simulink model "model"  (R2014a)
(part 5 of 5)

  powergui : powerlib/powergui  Priority=1  SimulationMode=Continuous  SolverType=Tustin  SampleTime=50e-6  frequency=60  SPID=off  DisableSnubberDevices=off  DisableRonSwitches=off  DisableVfSwitches=off  SwTol=0  Interpol=off  DisplayEquations=off  Ts=0  methode=off  frequencyindice=60  Pbase=100e6  ErrMax=1e-4  Iterations=50  UnitsV=kV  UnitsW=MW  FunctionMessages=off  echomessages=off  HookPort=off  EnableUseOfTLC=off  x0status=blocks  RestoreLinks=warning  ResistiveCurrentMeasurement=off  Frange=[0:2:500]  Ylog=off  Xlog=on  ShowGrid=off  save=off  variable=ZData  structure=0  ZoomFFT=off  StartTime=0.0  cycles=1  DisplayStyle=1  fundamental=60  FreqAxis=off  MaxFrequency=1000  frequencyindicesteady=1  RmsSteady=1  display=off
  Ötztal___Zirl_CN_147563007_110000_CN_100404264_110000 : powerlib/Elements/Distributed Parameters Line  Phases=3  Frequency=60  Resistance=[0.01273 0.3864]  Inductance="[0.9337e-3  4.1264e-3]"  Capacitance=[12.74e-9 7.751e-9]  Length=100  x1=[0 0 0 0; 0.0001244 0 0 0; 0.0002488 0 0 0; 0.0003733 0 0 0; 0.0004977 0 0 0; 0.0006221 0 0 0]  x2=[0 0 0 0; 0.0001244 0 0 0; 0.0002488 0 0 0; 0.0003733 0 0 0; 0.0004977 0 0 0; 0.0006221 0 0 0]  x3=[0 0 0 0; 0.0001244 0 0 0; 0.0002488 0 0 0; 0.0003733 0 0 0; 0.0004977 0 0 0; 0.0006221 0 0 0]  x4=[0 0 0 0; 0.0001244 0 0 0; 0.0002488 0 0 0; 0.0003733 0 0 0; 0.0004977 0 0 0; 0.0006221 0 0 0]  x5=0  V1=ones(3,3)  V2=ones(3,3)  I1=ones(3,3)  I2=ones(3,3)  nHarmo=1  Measurements=None
  connections:
  _CN_403466241_230000_CN_403481611_230000/LConn1 -- T_403466241__/LConn1 -- _CN_403466241_230000_CN_401936547_230000/LConn1
  _CN_403466241_230000_CN_403481611_230000/LConn2 -- T_403466241__/LConn2 -- _CN_403466241_230000_CN_401936547_230000/LConn2
  _CN_403466241_230000_CN_403481611_230000/LConn3 -- T_403466241__/LConn3 -- _CN_403466241_230000_CN_401936547_230000/LConn3 -- bus1/LConn1
  _CN_403466241_230000_CN_403481611_230000/RConn1 -- T_403481611__/LConn1 -- _CN_403481611_230000_CN_252757805_230000/LConn1 -- _CN_403481611_230000_CN_381823435_230000/LConn1
  _CN_403466241_230000_CN_403481611_230000/RConn2 -- T_403481611__/LConn2 -- _CN_403481611_230000_CN_252757805_230000/LConn2 -- _CN_403481611_230000_CN_381823435_230000/LConn2
  _CN_403466241_230000_CN_403481611_230000/RConn3 -- T_403481611__/LConn3 -- _CN_403481611_230000_CN_252757805_230000/LConn3 -- bus2/LConn1 -- _CN_403481611_230000_CN_381823435_230000/LConn3
  _CN_403466241_230000_CN_401936547_230000/RConn1 -- T_401936547__/RConn1 -- _CN_401936547_230000_CN_254460966_230000/LConn1 -- _CN_401936547_230000_CN_403504849_230000/LConn1 -- L_401936547/LConn1
  _CN_403466241_230000_CN_401936547_230000/RConn2 -- T_401936547__/RConn2 -- _CN_401936547_230000_CN_254460966_230000/LConn2 -- _CN_401936547_230000_CN_403504849_230000/LConn2 -- L_401936547/LConn2
  _CN_403466241_230000_CN_401936547_230000/RConn3 -- T_401936547__/RConn3 -- _CN_401936547_230000_CN_254460966_230000/LConn3 -- _CN_401936547_230000_CN_403504849_230000/LConn3 -- L_401936547/LConn3 -- bus3/LConn1
  _CN_404544820_230000_CN_404544831_230000/LConn1 -- T_404544820__/LConn1 -- _CN_404544820_230000_CN_107789748_230000/LConn1
  _CN_404544820_230000_CN_404544831_230000/LConn2 -- T_404544820__/LConn2 -- _CN_404544820_230000_CN_107789748_230000/LConn2
  _CN_404544820_230000_CN_404544831_230000/LConn3 -- T_404544820__/LConn3 -- _CN_404544820_230000_CN_107789748_230000/LConn3 -- bus4/LConn1
  T_404544831__/LConn1 -- _CN_404544820_230000_CN_404544831_230000/RConn1
  T_404544831__/LConn2 -- _CN_404544820_230000_CN_404544831_230000/RConn2
  _CN_404544820_230000_CN_404544831_230000/RConn3 -- T_404544831__/LConn3 -- bus5/LConn1
  _CN_404544820_230000_CN_107789748_230000/RConn1 -- G_107789748_/RConn1 -- _CN_403525677_230000_CN_107789748_230000/LConn1 -- _CN_296560688_230000_CN_107789748_230000/LConn1
  _CN_404544820_230000_CN_107789748_230000/RConn2 -- G_107789748_/RConn2 -- _CN_403525677_230000_CN_107789748_230000/LConn2 -- _CN_296560688_230000_CN_107789748_230000/LConn2
  _CN_404544820_230000_CN_107789748_230000/RConn3 -- G_107789748_/RConn3 -- _CN_403525677_230000_CN_107789748_230000/LConn3 -- _CN_296560688_230000_CN_107789748_230000/LConn3 -- bus6/LConn1
  _CN_407739530_230000_CN_195977249_230000/LConn1 -- T_407739530__/LConn1 -- _CN_407739530_230000_CN_199773788_230000/LConn1
  _CN_407739530_230000_CN_195977249_230000/LConn2 -- T_407739530__/LConn2 -- _CN_407739530_230000_CN_199773788_230000/LConn2
  _CN_407739530_230000_CN_195977249_230000/LConn3 -- T_407739530__/LConn3 -- _CN_407739530_230000_CN_199773788_230000/LConn3 -- bus7/LConn1
  _CN_407739530_230000_CN_195977249_230000/RConn1 -- T_195977249__สถานีไฟฟ้าแรงสูง_นครชัยศรี/LConn1 -- _CN_195977249_230000_CN_133318523_230000/LConn1
  _CN_407739530_230000_CN_195977249_230000/RConn2 -- T_195977249__สถานีไฟฟ้าแรงสูง_นครชัยศรี/LConn2 -- _CN_195977249_230000_CN_133318523_230000/LConn2
  _CN_407739530_230000_CN_195977249_230000/RConn3 -- T_195977249__สถานีไฟฟ้าแรงสูง_นครชัยศรี/LConn3 -- _CN_195977249_230000_CN_133318523_230000/LConn3 -- bus8/LConn1
  _CN_407739530_230000_CN_199773788_230000/RConn1 -- T_199773788__/LConn1 -- _CN_199773777_230000_CN_199773788_230000/LConn1 -- _CN_199773788_230000_CN_387737843_230000/LConn1 -- _CN_199773788_230000_CN_232344443_230000/LConn1 -- _CN_334185872_230000_CN_199773788_230000/LConn1
  _CN_407739530_230000_CN_199773788_230000/RConn2 -- T_199773788__/LConn2 -- _CN_199773777_230000_CN_199773788_230000/LConn2 -- _CN_199773788_230000_CN_387737843_230000/LConn2 -- _CN_199773788_230000_CN_232344443_230000/LConn2 -- _CN_334185872_230000_CN_199773788_230000/LConn2
  _CN_407739530_230000_CN_199773788_230000/RConn3 -- T_199773788__/LConn3 -- _CN_199773777_230000_CN_199773788_230000/LConn3 -- _CN_199773788_230000_CN_387737843_230000/LConn3 -- _CN_199773788_230000_CN_232344443_230000/LConn3 -- bus9/LConn1 -- _CN_334185872_230000_CN_199773788_230000/LConn3
  _CN_403481611_230000_CN_381823435_230000/RConn1 -- T_381823435__/LConn1 -- _CN_404563246_230000_CN_381823435_230000/LConn1
  _CN_403481611_230000_CN_381823435_230000/RConn2 -- T_381823435__/LConn2 -- _CN_404563246_230000_CN_381823435_230000/LConn2
  _CN_403481611_230000_CN_381823435_230000/RConn3 -- T_381823435__/LConn3 -- _CN_404563246_230000_CN_381823435_230000/LConn3 -- bus10/LConn1
  _CN_403481611_230000_CN_252757805_230000/RConn1 -- T_252757805__/LConn1 -- _CN_254460966_230000_CN_252757805_230000/LConn1
  _CN_403481611_230000_CN_252757805_230000/RConn2 -- T_252757805__/LConn2 -- _CN_254460966_230000_CN_252757805_230000/LConn2
  _CN_403481611_230000_CN_252757805_230000/RConn3 -- T_252757805__/LConn3 -- _CN_254460966_230000_CN_252757805_230000/LConn3 -- bus11/LConn1
  T_403525677__/LConn1 -- _CN_403525677_230000_CN_107789748_230000/RConn1
  T_403525677__/LConn2 -- _CN_403525677_230000_CN_107789748_230000/RConn2
  _CN_403525677_230000_CN_107789748_230000/RConn3 -- T_403525677__/LConn3 -- bus12/LConn1
  _CN_334185872_230000_CN_262815047_230000/LConn1 -- T_334185872__/LConn1 -- _CN_334185872_230000_CN_199773788_230000/RConn1
  _CN_334185872_230000_CN_262815047_230000/LConn2 -- T_334185872__/LConn2 -- _CN_334185872_230000_CN_199773788_230000/RConn2
  _CN_334185872_230000_CN_262815047_230000/LConn3 -- T_334185872__/LConn3 -- _CN_334185872_230000_CN_199773788_230000/RConn3 -- bus13/LConn1
  T_262815047__/LConn1 -- _CN_334185872_230000_CN_262815047_230000/RConn1
  T_262815047__/LConn2 -- _CN_334185872_230000_CN_262815047_230000/RConn2
  _CN_334185872_230000_CN_262815047_230000/RConn3 -- T_262815047__/LConn3 -- bus14/LConn1
  T_404006545__/LConn1 -- _CN_404006545_230000_CN_403692059_230000/LConn1
  T_404006545__/LConn2 -- _CN_404006545_230000_CN_403692059_230000/LConn2
  _CN_404006545_230000_CN_403692059_230000/LConn3 -- T_404006545__/LConn3 -- bus15/LConn1
  _CN_404006545_230000_CN_403692059_230000/RConn1 -- T_403692059__/LConn1 -- _CN_223601302_230000_CN_403692059_230000/LConn1 -- _CN_403692059_230000_CN_155851424_230000/LConn1
  _CN_404006545_230000_CN_403692059_230000/RConn2 -- T_403692059__/LConn2 -- _CN_223601302_230000_CN_403692059_230000/LConn2 -- _CN_403692059_230000_CN_155851424_230000/LConn2
  _CN_404006545_230000_CN_403692059_230000/RConn3 -- T_403692059__/LConn3 -- _CN_223601302_230000_CN_403692059_230000/LConn3 -- _CN_403692059_230000_CN_155851424_230000/LConn3 -- bus16/LConn1
  _CN_250742034_230000_CN_388836605_230000/LConn1 -- T_250742034__/RConn1 -- L_250742034/LConn1
  _CN_250742034_230000_CN_388836605_230000/LConn2 -- T_250742034__/RConn2 -- L_250742034/LConn2
  _CN_250742034_230000_CN_388836605_230000/LConn3 -- T_250742034__/RConn3 -- L_250742034/LConn3 -- bus17/LConn1
  _CN_250742034_230000_CN_388836605_230000/RConn1 -- T_388836605_230000_/LConn1 -- _CN_234182441_230000_CN_388836605_230000/LConn1
  _CN_250742034_230000_CN_388836605_230000/RConn2 -- T_388836605_230000_/LConn2 -- _CN_234182441_230000_CN_388836605_230000/LConn2
  _CN_250742034_230000_CN_388836605_230000/RConn3 -- T_388836605_230000_/LConn3 -- _CN_234182441_230000_CN_388836605_230000/LConn3 -- bus18/LConn1
  T_404291501__/LConn1 -- _CN_404291501_230000_CN_155851424_230000/LConn1
  T_404291501__/LConn2 -- _CN_404291501_230000_CN_155851424_230000/LConn2
  _CN_404291501_230000_CN_155851424_230000/LConn3 -- T_404291501__/LConn3 -- bus19/LConn1
  _CN_404291501_230000_CN_155851424_230000/RConn1 -- G_155851424_Bang_Pakong_Power_Plant/RConn1 -- _CN_345996520_230000_CN_155851424_230000/LConn1 -- _CN_404291513_230000_CN_155851424_230000/LConn1 -- _CN_223601302_230000_CN_155851424_230000/LConn1 -- _CN_403692059_230000_CN_155851424_230000/RConn1
  _CN_404291501_230000_CN_155851424_230000/RConn2 -- G_155851424_Bang_Pakong_Power_Plant/RConn2 -- _CN_345996520_230000_CN_155851424_230000/LConn2 -- _CN_404291513_230000_CN_155851424_230000/LConn2 -- _CN_223601302_230000_CN_155851424_230000/LConn2 -- _CN_403692059_230000_CN_155851424_230000/RConn2
  _CN_404291501_230000_CN_155851424_230000/RConn3 -- G_155851424_Bang_Pakong_Power_Plant/RConn3 -- _CN_345996520_230000_CN_155851424_230000/LConn3 -- bus20/LConn1 -- _CN_404291513_230000_CN_155851424_230000/LConn3 -- _CN_223601302_230000_CN_155851424_230000/LConn3 -- _CN_403692059_230000_CN_155851424_230000/RConn3
  _CN_404563246_230000_CN_176322698_230000/LConn1 -- T_404563246__/LConn1 -- _CN_404563246_230000_CN_404572911_230000/LConn1 -- _CN_404563246_230000_CN_381823435_230000/RConn1
  _CN_404563246_230000_CN_176322698_230000/LConn2 -- T_404563246__/LConn2 -- _CN_404563246_230000_CN_404572911_230000/LConn2 -- _CN_404563246_230000_CN_381823435_230000/RConn2
  _CN_404563246_230000_CN_176322698_230000/LConn3 -- T_404563246__/LConn3 -- _CN_404563246_230000_CN_404572911_230000/LConn3 -- bus21/LConn1 -- _CN_404563246_230000_CN_381823435_230000/RConn3
  _CN_404563246_230000_CN_176322698_230000/RConn1 -- G_176322698_Wang_Noi_Power_Station/RConn1 -- _CN_381823390_230000_CN_176322698_230000/LConn1 -- _CN_401936547_500000_CN_176322698_230000/LConn1 -- _CN_261489769_500000_CN_176322698_230000/LConn1 -- _CN_155847885_500000_CN_176322698_230000/LConn1 -- _CN_199773777_500000_CN_176322698_230000/LConn1 -- _CN_223601302_500000_CN_176322698_230000/LConn1 -- _CN_381823390_500000_CN_176322698_230000/LConn1
  _CN_404563246_230000_CN_176322698_230000/RConn2 -- G_176322698_Wang_Noi_Power_Station/RConn2 -- _CN_381823390_230000_CN_176322698_230000/LConn2 -- _CN_401936547_500000_CN_176322698_230000/LConn2 -- _CN_261489769_500000_CN_176322698_230000/LConn2 -- _CN_155847885_500000_CN_176322698_230000/LConn2 -- _CN_199773777_500000_CN_176322698_230000/LConn2 -- _CN_223601302_500000_CN_176322698_230000/LConn2 -- _CN_381823390_500000_CN_176322698_230000/LConn2
  _CN_404563246_230000_CN_176322698_230000/RConn3 -- G_176322698_Wang_Noi_Power_Station/RConn3 -- _CN_381823390_230000_CN_176322698_230000/LConn3 -- _CN_401936547_500000_CN_176322698_230000/LConn3 -- _CN_261489769_500000_CN_176322698_230000/LConn3 -- _CN_155847885_500000_CN_176322698_230000/LConn3 -- _CN_199773777_500000_CN_176322698_230000/LConn3 -- _CN_223601302_500000_CN_176322698_230000/LConn3 -- _CN_381823390_500000_CN_176322698_230000/LConn3 -- bus22/LConn1
  G_404572911_/RConn1 -- _CN_404563246_230000_CN_404572911_230000/RConn1
  G_404572911_/RConn2 -- _CN_404563246_230000_CN_404572911_230000/RConn2
  _CN_404563246_230000_CN_404572911_230000/RConn3 -- G_404572911_/RConn3 -- bus23/LConn1
  _CN_223601302_230000_CN_403692059_230000/RConn1 -- T_223601302__/RConn1 -- _CN_223601302_230000_CN_155851424_230000/RConn1 -- _CN_223601302_230000_CN_156592382_230000/LConn1 -- _CN_223601302_230000_CN_27828836_230000/LConn1 -- L_223601302/LConn1
  _CN_223601302_230000_CN_403692059_230000/RConn2 -- T_223601302__/RConn2 -- _CN_223601302_230000_CN_155851424_230000/RConn2 -- _CN_223601302_230000_CN_156592382_230000/LConn2 -- _CN_223601302_230000_CN_27828836_230000/LConn2 -- L_223601302/LConn2
  _CN_223601302_230000_CN_403692059_230000/RConn3 -- T_223601302__/RConn3 -- _CN_223601302_230000_CN_155851424_230000/RConn3 -- _CN_223601302_230000_CN_156592382_230000/LConn3 -- _CN_223601302_230000_CN_27828836_230000/LConn3 -- L_223601302/LConn3 -- bus24/LConn1
  _CN_223601302_230000_CN_156592382_230000/RConn1 -- T_156592382__/LConn1 -- _CN_404291513_230000_CN_156592382_230000/LConn1
  _CN_223601302_230000_CN_156592382_230000/RConn2 -- T_156592382__/LConn2 -- _CN_404291513_230000_CN_156592382_230000/LConn2
  _CN_223601302_230000_CN_156592382_230000/RConn3 -- T_156592382__/LConn3 -- _CN_404291513_230000_CN_156592382_230000/LConn3 -- bus25/LConn1
  _CN_223601302_230000_CN_27828836_230000/RConn1 -- T_27828836_230000_/LConn1 -- _CN_199773777_230000_CN_27828836_230000/LConn1 -- _CN_381823390_230000_CN_27828836_230000/LConn1 -- _CN_26238367_230000_CN_27828836_230000/LConn1
  _CN_223601302_230000_CN_27828836_230000/RConn2 -- T_27828836_230000_/LConn2 -- _CN_199773777_230000_CN_27828836_230000/LConn2 -- _CN_381823390_230000_CN_27828836_230000/LConn2 -- _CN_26238367_230000_CN_27828836_230000/LConn2
  _CN_223601302_230000_CN_27828836_230000/RConn3 -- T_27828836_230000_/LConn3 -- _CN_199773777_230000_CN_27828836_230000/LConn3 -- bus26/LConn1 -- _CN_381823390_230000_CN_27828836_230000/LConn3 -- _CN_26238367_230000_CN_27828836_230000/LConn3
  _CN_147606553_230000_CN_199773777_230000/LConn1 -- T_147606553_230000_/LConn1 -- _CN_147606553_230000_CN_199806286_230000/LConn1 -- _CN_147606553_230000_CN_408050988_230000/LConn1 -- _CN_147606553_230000_CN_301623867_230000/LConn1 -- _CN_147606553_230000_CN_26120059_230000/LConn1
  _CN_147606553_230000_CN_199773777_230000/LConn2 -- T_147606553_230000_/LConn2 -- _CN_147606553_230000_CN_199806286_230000/LConn2 -- _CN_147606553_230000_CN_408050988_230000/LConn2 -- _CN_147606553_230000_CN_301623867_230000/LConn2 -- _CN_147606553_230000_CN_26120059_230000/LConn2
  _CN_147606553_230000_CN_199773777_230000/LConn3 -- T_147606553_230000_/LConn3 -- _CN_147606553_230000_CN_199806286_230000/LConn3 -- _CN_147606553_230000_CN_408050988_230000/LConn3 -- _CN_147606553_230000_CN_301623867_230000/LConn3 -- _CN_147606553_230000_CN_26120059_230000/LConn3 -- bus27/LConn1
  _CN_147606553_230000_CN_199773777_230000/RConn1 -- T_199773777_500000;230000_/RConn1 -- _CN_199773777_230000_CN_199773788_230000/RConn1 -- L_199773777/LConn1 -- _CN_199773777_230000_CN_27828836_230000/RConn1
  _CN_147606553_230000_CN_199773777_230000/RConn2 -- T_199773777_500000;230000_/RConn2 -- _CN_199773777_230000_CN_199773788_230000/RConn2 -- L_199773777/LConn2 -- _CN_199773777_230000_CN_27828836_230000/RConn2
  _CN_147606553_230000_CN_199773777_230000/RConn3 -- T_199773777_500000;230000_/RConn3 -- _CN_199773777_230000_CN_199773788_230000/RConn3 -- L_199773777/LConn3 -- bus28/LConn1 -- _CN_199773777_230000_CN_27828836_230000/RConn3
  _CN_147606553_230000_CN_199806286_230000/RConn1 -- T_199806286__/LConn1 -- _CN_26238367_230000_CN_199806286_230000/LConn1
  _CN_147606553_230000_CN_199806286_230000/RConn2 -- T_199806286__/LConn2 -- _CN_26238367_230000_CN_199806286_230000/LConn2
  _CN_147606553_230000_CN_199806286_230000/RConn3 -- T_199806286__/LConn3 -- _CN_26238367_230000_CN_199806286_230000/LConn3 -- bus29/LConn1
  _CN_147606553_230000_CN_408050988_230000/RConn1 -- T_408050988__/LConn1 -- _CN_408050988_230000_CN_133318523_230000/LConn1
  _CN_147606553_230000_CN_408050988_230000/RConn2 -- T_408050988__/LConn2 -- _CN_408050988_230000_CN_133318523_230000/LConn2
  _CN_147606553_230000_CN_408050988_230000/RConn3 -- T_408050988__/LConn3 -- _CN_408050988_230000_CN_133318523_230000/LConn3 -- bus30/LConn1
  T_301623867__สถานีไฟฟ้าแรงสูง_ธนบุรีใต้/LConn1 -- _CN_147606553_230000_CN_301623867_230000/RConn1
  T_301623867__สถานีไฟฟ้าแรงสูง_ธนบุรีใต้/LConn2 -- _CN_147606553_230000_CN_301623867_230000/RConn2
  _CN_147606553_230000_CN_301623867_230000/RConn3 -- T_301623867__สถานีไฟฟ้าแรงสูง_ธนบุรีใต้/LConn3 -- bus31/LConn1
  _CN_147606553_230000_CN_26120059_230000/RConn1 -- T_26120059_230000_/LConn1 -- _CN_64680223_230000_CN_26120059_230000/LConn1
  _CN_147606553_230000_CN_26120059_230000/RConn2 -- T_26120059_230000_/LConn2 -- _CN_64680223_230000_CN_26120059_230000/LConn2
  _CN_147606553_230000_CN_26120059_230000/RConn3 -- T_26120059_230000_/LConn3 -- _CN_64680223_230000_CN_26120059_230000/LConn3 -- bus32/LConn1
  T_295988731__Chana/LConn1 -- _CN_295988731_230000_CN_244062167_230000/LConn1
  T_295988731__Chana/LConn2 -- _CN_295988731_230000_CN_244062167_230000/LConn2
  _CN_295988731_230000_CN_244062167_230000/LConn3 -- T_295988731__Chana/LConn3 -- bus33/LConn1
  _CN_295988731_230000_CN_244062167_230000/RConn1 -- T_244062167__/LConn1 -- _CN_324258748_230000_CN_244062167_230000/LConn1
  _CN_295988731_230000_CN_244062167_230000/RConn2 -- T_244062167__/LConn2 -- _CN_324258748_230000_CN_244062167_230000/LConn2
  _CN_295988731_230000_CN_244062167_230000/RConn3 -- T_244062167__/LConn3 -- _CN_324258748_230000_CN_244062167_230000/LConn3 -- bus34/LConn1
  _CN_381823390_230000_CN_176322698_230000/RConn1 -- T_381823390_500000;230000_/RConn1 -- _CN_381823390_230000_CN_403512774_230000/LConn1 -- _CN_381823390_230000_CN_27828836_230000/RConn1 -- L_381823390/LConn1
  _CN_381823390_230000_CN_176322698_230000/RConn2 -- T_381823390_500000;230000_/RConn2 -- _CN_381823390_230000_CN_403512774_230000/LConn2 -- _CN_381823390_230000_CN_27828836_230000/RConn2 -- L_381823390/LConn2
  _CN_381823390_230000_CN_176322698_230000/RConn3 -- T_381823390_500000;230000_/RConn3 -- _CN_381823390_230000_CN_403512774_230000/LConn3 -- _CN_381823390_230000_CN_27828836_230000/RConn3 -- L_381823390/LConn3 -- bus35/LConn1
  _CN_381823390_230000_CN_403512774_230000/RConn1 -- T_403512774__/LConn1 -- _CN_403512774_230000_CN_403504849_230000/LConn1
  _CN_381823390_230000_CN_403512774_230000/RConn2 -- T_403512774__/LConn2 -- _CN_403512774_230000_CN_403504849_230000/LConn2
  _CN_381823390_230000_CN_403512774_230000/RConn3 -- T_403512774__/LConn3 -- _CN_403512774_230000_CN_403504849_230000/LConn3 -- bus36/LConn1
  _CN_26238367_230000_CN_27828836_230000/RConn1 -- T_26238367__/LConn1 -- _CN_26238367_230000_CN_274223991_230000/LConn1 -- _CN_26238367_230000_CN_199806286_230000/RConn1
  _CN_26238367_230000_CN_27828836_230000/RConn2 -- T_26238367__/LConn2 -- _CN_26238367_230000_CN_274223991_230000/LConn2 -- _CN_26238367_230000_CN_199806286_230000/RConn2
  _CN_26238367_230000_CN_27828836_230000/RConn3 -- T_26238367__/LConn3 -- _CN_26238367_230000_CN_274223991_230000/LConn3 -- _CN_26238367_230000_CN_199806286_230000/RConn3 -- bus37/LConn1
  _CN_26238367_230000_CN_274223991_230000/RConn1 -- T_274223991__/LConn1 -- _CN_274223991_230000_CN_64680159_230000/LConn1
  _CN_26238367_230000_CN_274223991_230000/RConn2 -- T_274223991__/LConn2 -- _CN_274223991_230000_CN_64680159_230000/LConn2
  _CN_26238367_230000_CN_274223991_230000/RConn3 -- T_274223991__/LConn3 -- _CN_274223991_230000_CN_64680159_230000/LConn3 -- bus38/LConn1
  _CN_195977249_230000_CN_133318523_230000/RConn1 -- T_133318523__/LConn1 -- _CN_408050988_230000_CN_133318523_230000/RConn1
  _CN_195977249_230000_CN_133318523_230000/RConn2 -- T_133318523__/LConn2 -- _CN_408050988_230000_CN_133318523_230000/RConn2
  _CN_195977249_230000_CN_133318523_230000/RConn3 -- T_133318523__/LConn3 -- _CN_408050988_230000_CN_133318523_230000/RConn3 -- bus39/LConn1
  _CN_401936547_230000_CN_254460966_230000/RConn1 -- T_254460966__/LConn1 -- _CN_254460966_230000_CN_401998847_230000/LConn1 -- _CN_254460966_230000_CN_252757805_230000/RConn1
  _CN_401936547_230000_CN_254460966_230000/RConn2 -- T_254460966__/LConn2 -- _CN_254460966_230000_CN_401998847_230000/LConn2 -- _CN_254460966_230000_CN_252757805_230000/RConn2
  _CN_401936547_230000_CN_254460966_230000/RConn3 -- T_254460966__/LConn3 -- _CN_254460966_230000_CN_401998847_230000/LConn3 -- _CN_254460966_230000_CN_252757805_230000/RConn3 -- bus40/LConn1
  _CN_401936547_230000_CN_403504849_230000/RConn1 -- T_403504849__/LConn1 -- _CN_403512774_230000_CN_403504849_230000/RConn1
  _CN_401936547_230000_CN_403504849_230000/RConn2 -- T_403504849__/LConn2 -- _CN_403512774_230000_CN_403504849_230000/RConn2
  _CN_401936547_230000_CN_403504849_230000/RConn3 -- T_403504849__/LConn3 -- _CN_403512774_230000_CN_403504849_230000/RConn3 -- bus41/LConn1
  _CN_254460966_230000_CN_401998847_230000/RConn1 -- T_401998847__/LConn1 -- _CN_384684882_230000_CN_401998847_230000/LConn1
  _CN_254460966_230000_CN_401998847_230000/RConn2 -- T_401998847__/LConn2 -- _CN_384684882_230000_CN_401998847_230000/LConn2
  _CN_254460966_230000_CN_401998847_230000/RConn3 -- T_401998847__/LConn3 -- _CN_384684882_230000_CN_401998847_230000/LConn3 -- bus42/LConn1
  T_382334119_500000;230000_/LConn1 -- _CN_382334119_230000_CN_247878196_230000/LConn1
  T_382334119_500000;230000_/LConn2 -- _CN_382334119_230000_CN_247878196_230000/LConn2
  _CN_382334119_230000_CN_247878196_230000/LConn3 -- T_382334119_500000;230000_/LConn3 -- bus43/LConn1
  T_247878196_230000;115000_/LConn1 -- _CN_382334119_230000_CN_247878196_230000/RConn1
  T_247878196_230000;115000_/LConn2 -- _CN_382334119_230000_CN_247878196_230000/RConn2
  _CN_382334119_230000_CN_247878196_230000/RConn3 -- T_247878196_230000;115000_/LConn3 -- bus44/LConn1
  T_234182441__/LConn1 -- _CN_234182441_230000_CN_388836605_230000/RConn1
  T_234182441__/LConn2 -- _CN_234182441_230000_CN_388836605_230000/RConn2
  _CN_234182441_230000_CN_388836605_230000/RConn3 -- T_234182441__/LConn3 -- bus45/LConn1
  T_408425007__/LConn1 -- _CN_408425007_230000_CN_387737843_230000/LConn1
  T_408425007__/LConn2 -- _CN_408425007_230000_CN_387737843_230000/LConn2
  _CN_408425007_230000_CN_387737843_230000/LConn3 -- T_408425007__/LConn3 -- bus46/LConn1
  _CN_408425007_230000_CN_387737843_230000/RConn1 -- T_387737843__/LConn1 -- _CN_199773788_230000_CN_387737843_230000/RConn1
  _CN_408425007_230000_CN_387737843_230000/RConn2 -- T_387737843__/LConn2 -- _CN_199773788_230000_CN_387737843_230000/RConn2
  _CN_408425007_230000_CN_387737843_230000/RConn3 -- T_387737843__/LConn3 -- _CN_199773788_230000_CN_387737843_230000/RConn3 -- bus47/LConn1
  _CN_296560688_230000_CN_107789748_230000/RConn1 -- T_296560688__/LConn1 -- _CN_296560688_230000_CN_155847885_230000/LConn1
  _CN_296560688_230000_CN_107789748_230000/RConn2 -- T_296560688__/LConn2 -- _CN_296560688_230000_CN_155847885_230000/LConn2
  _CN_296560688_230000_CN_107789748_230000/RConn3 -- T_296560688__/LConn3 -- _CN_296560688_230000_CN_155847885_230000/LConn3 -- bus48/LConn1
  _CN_296560688_230000_CN_155847885_230000/RConn1 -- T_155847885__/RConn1 -- L_155847885/LConn1
  _CN_296560688_230000_CN_155847885_230000/RConn2 -- T_155847885__/RConn2 -- L_155847885/LConn2
  _CN_296560688_230000_CN_155847885_230000/RConn3 -- T_155847885__/RConn3 -- L_155847885/LConn3 -- bus49/LConn1
  _CN_404291513_230000_CN_156592382_230000/RConn1 -- T_404291513__/LConn1 -- _CN_404291513_230000_CN_155851424_230000/RConn1
  _CN_404291513_230000_CN_156592382_230000/RConn2 -- T_404291513__/LConn2 -- _CN_404291513_230000_CN_155851424_230000/RConn2
  _CN_404291513_230000_CN_156592382_230000/RConn3 -- T_404291513__/LConn3 -- _CN_404291513_230000_CN_155851424_230000/RConn3 -- bus50/LConn1
  _CN_64680223_230000_CN_345996520_230000/LConn1 -- T_64680223_230000_/LConn1 -- _CN_64680223_230000_CN_26120059_230000/RConn1
  _CN_64680223_230000_CN_345996520_230000/LConn2 -- T_64680223_230000_/LConn2 -- _CN_64680223_230000_CN_26120059_230000/RConn2
  _CN_64680223_230000_CN_345996520_230000/LConn3 -- T_64680223_230000_/LConn3 -- _CN_64680223_230000_CN_26120059_230000/RConn3 -- bus51/LConn1
  _CN_64680223_230000_CN_345996520_230000/RConn1 -- T_345996520__/LConn1 -- _CN_345996520_230000_CN_155851424_230000/RConn1 -- _CN_345996520_230000_CN_64680187_230000/LConn1
  _CN_64680223_230000_CN_345996520_230000/RConn2 -- T_345996520__/LConn2 -- _CN_345996520_230000_CN_155851424_230000/RConn2 -- _CN_345996520_230000_CN_64680187_230000/LConn2
  _CN_64680223_230000_CN_345996520_230000/RConn3 -- T_345996520__/LConn3 -- _CN_345996520_230000_CN_155851424_230000/RConn3 -- bus52/LConn1 -- _CN_345996520_230000_CN_64680187_230000/LConn3
  T_324258748__HVDC_Thai__Mal/LConn1 -- _CN_324258748_230000_CN_244062167_230000/RConn1
  T_324258748__HVDC_Thai__Mal/LConn2 -- _CN_324258748_230000_CN_244062167_230000/RConn2
  _CN_324258748_230000_CN_244062167_230000/RConn3 -- T_324258748__HVDC_Thai__Mal/LConn3 -- bus53/LConn1
  T_144455497__/LConn1 -- _CN_144455497_230000_CN_384689050_230000/LConn1
  T_144455497__/LConn2 -- _CN_144455497_230000_CN_384689050_230000/LConn2
  _CN_144455497_230000_CN_384689050_230000/LConn3 -- T_144455497__/LConn3 -- bus54/LConn1
  _CN_144455497_230000_CN_384689050_230000/RConn1 -- G_384689050_/RConn1 -- _CN_384684882_230000_CN_384689050_230000/LConn1 -- _CN_293324904_230000_CN_384689050_230000/LConn1 -- _CN_401936547_500000_CN_384689050_230000/LConn1
  _CN_144455497_230000_CN_384689050_230000/RConn2 -- G_384689050_/RConn2 -- _CN_384684882_230000_CN_384689050_230000/LConn2 -- _CN_293324904_230000_CN_384689050_230000/LConn2 -- _CN_401936547_500000_CN_384689050_230000/LConn2
  _CN_144455497_230000_CN_384689050_230000/RConn3 -- G_384689050_/RConn3 -- _CN_384684882_230000_CN_384689050_230000/LConn3 -- _CN_293324904_230000_CN_384689050_230000/LConn3 -- _CN_401936547_500000_CN_384689050_230000/LConn3 -- bus55/LConn1
  _CN_274223991_230000_CN_64680159_230000/RConn1 -- T_64680159__/LConn1 -- _CN_64680159_230000_CN_64680187_230000/LConn1
  _CN_274223991_230000_CN_64680159_230000/RConn2 -- T_64680159__/LConn2 -- _CN_64680159_230000_CN_64680187_230000/LConn2
  _CN_274223991_230000_CN_64680159_230000/RConn3 -- T_64680159__/LConn3 -- _CN_64680159_230000_CN_64680187_230000/LConn3 -- bus56/LConn1
  T_381850832_230000;115000_Phangnga/LConn1 -- _CN_381850832_230000_CN_381850842_230000/LConn1
  T_381850832_230000;115000_Phangnga/LConn2 -- _CN_381850832_230000_CN_381850842_230000/LConn2
  _CN_381850832_230000_CN_381850842_230000/LConn3 -- T_381850832_230000;115000_Phangnga/LConn3 -- bus57/LConn1
  T_381850842_230000;115000_Phuket_2/LConn1 -- _CN_381850832_230000_CN_381850842_230000/RConn1
  T_381850842_230000;115000_Phuket_2/LConn2 -- _CN_381850832_230000_CN_381850842_230000/RConn2
  _CN_381850832_230000_CN_381850842_230000/RConn3 -- T_381850842_230000;115000_Phuket_2/LConn3 -- bus58/LConn1
  _CN_384684882_230000_CN_401998847_230000/RConn1 -- T_384684882__/LConn1 -- _CN_384684882_230000_CN_384689050_230000/RConn1
  _CN_384684882_230000_CN_401998847_230000/RConn2 -- T_384684882__/LConn2 -- _CN_384684882_230000_CN_384689050_230000/RConn2
  _CN_384684882_230000_CN_401998847_230000/RConn3 -- T_384684882__/LConn3 -- _CN_384684882_230000_CN_384689050_230000/RConn3 -- bus59/LConn1
  _CN_199773788_230000_CN_232344443_230000/RConn1 -- G_232344443_โรงไฟฟ้าราชบุรี/RConn1 -- _CN_362353140_230000_CN_232344443_230000/LConn1 -- _CN_362353140_500000_CN_232344443_230000/LConn1
  _CN_199773788_230000_CN_232344443_230000/RConn2 -- G_232344443_โรงไฟฟ้าราชบุรี/RConn2 -- _CN_362353140_230000_CN_232344443_230000/LConn2 -- _CN_362353140_500000_CN_232344443_230000/LConn2
  _CN_199773788_230000_CN_232344443_230000/RConn3 -- G_232344443_โรงไฟฟ้าราชบุรี/RConn3 -- _CN_362353140_230000_CN_232344443_230000/LConn3 -- _CN_362353140_500000_CN_232344443_230000/LConn3 -- bus60/LConn1
  _CN_64680159_230000_CN_64680187_230000/RConn1 -- T_64680187__/RConn1 -- _CN_345996520_230000_CN_64680187_230000/RConn1 -- L_64680187/LConn1
  _CN_64680159_230000_CN_64680187_230000/RConn2 -- T_64680187__/RConn2 -- _CN_345996520_230000_CN_64680187_230000/RConn2 -- L_64680187/LConn2
  _CN_64680159_230000_CN_64680187_230000/RConn3 -- T_64680187__/RConn3 -- _CN_345996520_230000_CN_64680187_230000/RConn3 -- L_64680187/LConn3 -- bus61/LConn1
  T_293324904__/LConn1 -- _CN_293324904_230000_CN_384689050_230000/RConn1
  T_293324904__/LConn2 -- _CN_293324904_230000_CN_384689050_230000/RConn2
  _CN_293324904_230000_CN_384689050_230000/RConn3 -- T_293324904__/LConn3 -- bus62/LConn1
  _CN_362353140_230000_CN_232344443_230000/RConn1 -- T_362353140__/RConn1 -- L_362353140/LConn1
  _CN_362353140_230000_CN_232344443_230000/RConn2 -- T_362353140__/RConn2 -- L_362353140/LConn2
  _CN_362353140_230000_CN_232344443_230000/RConn3 -- T_362353140__/RConn3 -- L_362353140/LConn3 -- bus63/LConn1
  _CN_401936547_500000_CN_176322698_230000/RConn1 -- T_401936547__/LConn1 -- _CN_401936547_500000_CN_293324915_500000/LConn1 -- _CN_401936547_500000_CN_384689050_230000/RConn1 -- _CN_401936547_500000_CN_223601302_500000/LConn1
  _CN_401936547_500000_CN_176322698_230000/RConn2 -- T_401936547__/LConn2 -- _CN_401936547_500000_CN_293324915_500000/LConn2 -- _CN_401936547_500000_CN_384689050_230000/RConn2 -- _CN_401936547_500000_CN_223601302_500000/LConn2
  _CN_401936547_500000_CN_176322698_230000/RConn3 -- T_401936547__/LConn3 -- _CN_401936547_500000_CN_293324915_500000/LConn3 -- _CN_401936547_500000_CN_384689050_230000/RConn3 -- _CN_401936547_500000_CN_223601302_500000/LConn3 -- bus64/LConn1
  T_293324915__/LConn1 -- _CN_401936547_500000_CN_293324915_500000/RConn1
  T_293324915__/LConn2 -- _CN_401936547_500000_CN_293324915_500000/RConn2
  _CN_401936547_500000_CN_293324915_500000/RConn3 -- T_293324915__/LConn3 -- bus65/LConn1
  _CN_401936547_500000_CN_223601302_500000/RConn1 -- T_223601302__/LConn1 -- _CN_223601302_500000_CN_64680187_500000/LConn1 -- _CN_223601302_500000_CN_176322698_230000/RConn1 -- _CN_155847885_500000_CN_223601302_500000/LConn1
  _CN_401936547_500000_CN_223601302_500000/RConn2 -- T_223601302__/LConn2 -- _CN_223601302_500000_CN_64680187_500000/LConn2 -- _CN_223601302_500000_CN_176322698_230000/RConn2 -- _CN_155847885_500000_CN_223601302_500000/LConn2
  _CN_401936547_500000_CN_223601302_500000/RConn3 -- T_223601302__/LConn3 -- _CN_223601302_500000_CN_64680187_500000/LConn3 -- _CN_223601302_500000_CN_176322698_230000/RConn3 -- bus66/LConn1 -- _CN_155847885_500000_CN_223601302_500000/LConn3
  T_242402501__/LConn1 -- _CN_242402501_500000_CN_155847885_500000/LConn1
  T_242402501__/LConn2 -- _CN_242402501_500000_CN_155847885_500000/LConn2
  _CN_242402501_500000_CN_155847885_500000/LConn3 -- T_242402501__/LConn3 -- bus67/LConn1
  _CN_242402501_500000_CN_155847885_500000/RConn1 -- T_155847885__/LConn1 -- _CN_155847885_500000_CN_176322698_230000/RConn1 -- _CN_155847885_500000_CN_223601302_500000/RConn1
  _CN_242402501_500000_CN_155847885_500000/RConn2 -- T_155847885__/LConn2 -- _CN_155847885_500000_CN_176322698_230000/RConn2 -- _CN_155847885_500000_CN_223601302_500000/RConn2
  _CN_242402501_500000_CN_155847885_500000/RConn3 -- T_155847885__/LConn3 -- _CN_155847885_500000_CN_176322698_230000/RConn3 -- _CN_155847885_500000_CN_223601302_500000/RConn3 -- bus68/LConn1
  T_362353137__/LConn1 -- _CN_362353137_500000_CN_362353140_500000/LConn1
  T_362353137__/LConn2 -- _CN_362353137_500000_CN_362353140_500000/LConn2
  _CN_362353137_500000_CN_362353140_500000/LConn3 -- T_362353137__/LConn3 -- bus69/LConn1
  _CN_362353137_500000_CN_362353140_500000/RConn1 -- T_362353140__/LConn1 -- _CN_362353140_500000_CN_232344443_230000/RConn1 -- _CN_261489769_500000_CN_362353140_500000/LConn1
  _CN_362353137_500000_CN_362353140_500000/RConn2 -- T_362353140__/LConn2 -- _CN_362353140_500000_CN_232344443_230000/RConn2 -- _CN_261489769_500000_CN_362353140_500000/LConn2
  _CN_362353137_500000_CN_362353140_500000/RConn3 -- T_362353140__/LConn3 -- _CN_362353140_500000_CN_232344443_230000/RConn3 -- bus70/LConn1 -- _CN_261489769_500000_CN_362353140_500000/LConn3
  _CN_261489769_500000_CN_176322698_230000/RConn1 -- T_261489769_500000_/LConn1 -- _CN_261489769_500000_CN_199773777_500000/LConn1 -- _CN_261489769_500000_CN_362353140_500000/RConn1 -- _CN_261489769_500000_CN_250742034_500000/LConn1
  _CN_261489769_500000_CN_176322698_230000/RConn2 -- T_261489769_500000_/LConn2 -- _CN_261489769_500000_CN_199773777_500000/LConn2 -- _CN_261489769_500000_CN_362353140_500000/RConn2 -- _CN_261489769_500000_CN_250742034_500000/LConn2
  _CN_261489769_500000_CN_176322698_230000/RConn3 -- T_261489769_500000_/LConn3 -- _CN_261489769_500000_CN_199773777_500000/LConn3 -- _CN_261489769_500000_CN_362353140_500000/RConn3 -- _CN_261489769_500000_CN_250742034_500000/LConn3 -- bus71/LConn1
  _CN_261489769_500000_CN_199773777_500000/RConn1 -- T_199773777_500000;230000_/LConn1 -- _CN_199773777_500000_CN_176322698_230000/RConn1
  _CN_261489769_500000_CN_199773777_500000/RConn2 -- T_199773777_500000;230000_/LConn2 -- _CN_199773777_500000_CN_176322698_230000/RConn2
  _CN_261489769_500000_CN_199773777_500000/RConn3 -- T_199773777_500000;230000_/LConn3 -- _CN_199773777_500000_CN_176322698_230000/RConn3 -- bus72/LConn1
  T_250742034__/LConn1 -- _CN_261489769_500000_CN_250742034_500000/RConn1
  T_250742034__/LConn2 -- _CN_261489769_500000_CN_250742034_500000/RConn2
  _CN_261489769_500000_CN_250742034_500000/RConn3 -- T_250742034__/LConn3 -- bus73/LConn1
  T_64680187__/LConn1 -- _CN_223601302_500000_CN_64680187_500000/RConn1
  T_64680187__/LConn2 -- _CN_223601302_500000_CN_64680187_500000/RConn2
  _CN_223601302_500000_CN_64680187_500000/RConn3 -- T_64680187__/LConn3 -- bus74/LConn1
  T_381823390_500000;230000_/LConn1 -- _CN_381823390_500000_CN_176322698_230000/RConn1
  T_381823390_500000;230000_/LConn2 -- _CN_381823390_500000_CN_176322698_230000/RConn2
  _CN_381823390_500000_CN_176322698_230000/RConn3 -- T_381823390_500000;230000_/LConn3 -- bus75/LConn1
  T_403466241__/RConn1 -- L_403466241/LConn1
  T_403466241__/RConn2 -- L_403466241/LConn2
  L_403466241/LConn3 -- T_403466241__/RConn3 -- bus76/LConn1
  T_403481611__/RConn1 -- L_403481611/LConn1
  T_403481611__/RConn2 -- L_403481611/LConn2
  L_403481611/LConn3 -- T_403481611__/RConn3 -- bus77/LConn1
  T_404544820__/RConn1 -- L_404544820/LConn1
  T_404544820__/RConn2 -- L_404544820/LConn2
  L_404544820/LConn3 -- T_404544820__/RConn3 -- bus78/LConn1
  T_404544831__/RConn1 -- L_404544831/LConn1
  T_404544831__/RConn2 -- L_404544831/LConn2
  L_404544831/LConn3 -- T_404544831__/RConn3 -- bus79/LConn1
  T_407739530__/RConn1 -- L_407739530/LConn1
  T_407739530__/RConn2 -- L_407739530/LConn2
  L_407739530/LConn3 -- T_407739530__/RConn3 -- bus80/LConn1
  T_195977249__สถานีไฟฟ้าแรงสูง_นครชัยศรี/RConn1 -- L_195977249/LConn1
  T_195977249__สถานีไฟฟ้าแรงสูง_นครชัยศรี/RConn2 -- L_195977249/LConn2
  L_195977249/LConn3 -- T_195977249__สถานีไฟฟ้าแรงสูง_นครชัยศรี/RConn3 -- bus81/LConn1
  T_199773788__/RConn1 -- L_199773788/LConn1
  T_199773788__/RConn2 -- L_199773788/LConn2
  L_199773788/LConn3 -- T_199773788__/RConn3 -- bus82/LConn1
  T_381823435__/RConn1 -- L_381823435/LConn1
  T_381823435__/RConn2 -- L_381823435/LConn2
  L_381823435/LConn3 -- T_381823435__/RConn3 -- bus83/LConn1
  T_252757805__/RConn1 -- L_252757805/LConn1
  T_252757805__/RConn2 -- L_252757805/LConn2
  L_252757805/LConn3 -- T_252757805__/RConn3 -- bus84/LConn1
  T_403525677__/RConn1 -- L_403525677/LConn1
  T_403525677__/RConn2 -- L_403525677/LConn2
  L_403525677/LConn3 -- T_403525677__/RConn3 -- bus85/LConn1
  T_334185872__/RConn1 -- L_334185872/LConn1
  T_334185872__/RConn2 -- L_334185872/LConn2
  L_334185872/LConn3 -- T_334185872__/RConn3 -- bus86/LConn1
  T_262815047__/RConn1 -- L_262815047/LConn1
  T_262815047__/RConn2 -- L_262815047/LConn2
  L_262815047/LConn3 -- T_262815047__/RConn3 -- bus87/LConn1
  T_404006545__/RConn1 -- L_404006545/LConn1
  T_404006545__/RConn2 -- L_404006545/LConn2
  L_404006545/LConn3 -- T_404006545__/RConn3 -- bus88/LConn1
  T_403692059__/RConn1 -- L_403692059/LConn1
  T_403692059__/RConn2 -- L_403692059/LConn2
  L_403692059/LConn3 -- T_403692059__/RConn3 -- bus89/LConn1
  T_388836605_230000_/RConn1 -- L_388836605/LConn1
  T_388836605_230000_/RConn2 -- L_388836605/LConn2
  L_388836605/LConn3 -- T_388836605_230000_/RConn3 -- bus90/LConn1
  T_404291501__/RConn1 -- L_404291501/LConn1
  T_404291501__/RConn2 -- L_404291501/LConn2
  L_404291501/LConn3 -- T_404291501__/RConn3 -- bus91/LConn1
  T_404563246__/RConn1 -- L_404563246/LConn1
  T_404563246__/RConn2 -- L_404563246/LConn2
  L_404563246/LConn3 -- T_404563246__/RConn3 -- bus92/LConn1
  T_156592382__/RConn1 -- L_156592382/LConn1
  T_156592382__/RConn2 -- L_156592382/LConn2
  L_156592382/LConn3 -- T_156592382__/RConn3 -- bus93/LConn1
  T_27828836_230000_/RConn1 -- L_27828836/LConn1
  T_27828836_230000_/RConn2 -- L_27828836/LConn2
  L_27828836/LConn3 -- T_27828836_230000_/RConn3 -- bus94/LConn1
  T_147606553_230000_/RConn1 -- L_147606553/LConn1
  T_147606553_230000_/RConn2 -- L_147606553/LConn2
  L_147606553/LConn3 -- T_147606553_230000_/RConn3 -- bus95/LConn1
  T_199806286__/RConn1 -- L_199806286/LConn1
  T_199806286__/RConn2 -- L_199806286/LConn2
  L_199806286/LConn3 -- T_199806286__/RConn3 -- bus96/LConn1
  T_408050988__/RConn1 -- L_408050988/LConn1
  T_408050988__/RConn2 -- L_408050988/LConn2
  L_408050988/LConn3 -- T_408050988__/RConn3 -- bus97/LConn1
  T_301623867__สถานีไฟฟ้าแรงสูง_ธนบุรีใต้/RConn1 -- L_301623867/LConn1
  T_301623867__สถานีไฟฟ้าแรงสูง_ธนบุรีใต้/RConn2 -- L_301623867/LConn2
  L_301623867/LConn3 -- T_301623867__สถานีไฟฟ้าแรงสูง_ธนบุรีใต้/RConn3 -- bus98/LConn1
  T_26120059_230000_/RConn1 -- L_26120059/LConn1
  T_26120059_230000_/RConn2 -- L_26120059/LConn2
  L_26120059/LConn3 -- T_26120059_230000_/RConn3 -- bus99/LConn1
  T_295988731__Chana/RConn1 -- L_295988731/LConn1
  T_295988731__Chana/RConn2 -- L_295988731/LConn2
  L_295988731/LConn3 -- T_295988731__Chana/RConn3 -- bus100/LConn1
  T_244062167__/RConn1 -- L_244062167/LConn1
  T_244062167__/RConn2 -- L_244062167/LConn2
  L_244062167/LConn3 -- T_244062167__/RConn3 -- bus101/LConn1
  T_403512774__/RConn1 -- L_403512774/LConn1
  T_403512774__/RConn2 -- L_403512774/LConn2
  L_403512774/LConn3 -- T_403512774__/RConn3 -- bus102/LConn1
  T_26238367__/RConn1 -- L_26238367/LConn1
  T_26238367__/RConn2 -- L_26238367/LConn2
  L_26238367/LConn3 -- T_26238367__/RConn3 -- bus103/LConn1
  T_274223991__/RConn1 -- L_274223991/LConn1
  T_274223991__/RConn2 -- L_274223991/LConn2
  L_274223991/LConn3 -- T_274223991__/RConn3 -- bus104/LConn1
  T_133318523__/RConn1 -- L_133318523/LConn1
  T_133318523__/RConn2 -- L_133318523/LConn2
  L_133318523/LConn3 -- T_133318523__/RConn3 -- bus105/LConn1
  T_254460966__/RConn1 -- L_254460966/LConn1
  T_254460966__/RConn2 -- L_254460966/LConn2
  L_254460966/LConn3 -- T_254460966__/RConn3 -- bus106/LConn1
  T_403504849__/RConn1 -- L_403504849/LConn1
  T_403504849__/RConn2 -- L_403504849/LConn2
  L_403504849/LConn3 -- T_403504849__/RConn3 -- bus107/LConn1
  T_401998847__/RConn1 -- L_401998847/LConn1
  T_401998847__/RConn2 -- L_401998847/LConn2
  L_401998847/LConn3 -- T_401998847__/RConn3 -- bus108/LConn1
  T_382334119_500000;230000_/RConn1 -- L_382334119/LConn1
  T_382334119_500000;230000_/RConn2 -- L_382334119/LConn2
  L_382334119/LConn3 -- T_382334119_500000;230000_/RConn3 -- bus109/LConn1
  T_247878196_230000;115000_/RConn1 -- L_247878196/LConn1
  T_247878196_230000;115000_/RConn2 -- L_247878196/LConn2
  L_247878196/LConn3 -- T_247878196_230000;115000_/RConn3 -- bus110/LConn1
  T_234182441__/RConn1 -- L_234182441/LConn1
  T_234182441__/RConn2 -- L_234182441/LConn2
  L_234182441/LConn3 -- T_234182441__/RConn3 -- bus111/LConn1
  T_408425007__/RConn1 -- L_408425007/LConn1
  T_408425007__/RConn2 -- L_408425007/LConn2
  L_408425007/LConn3 -- T_408425007__/RConn3 -- bus112/LConn1
  T_387737843__/RConn1 -- L_387737843/LConn1
  T_387737843__/RConn2 -- L_387737843/LConn2
  L_387737843/LConn3 -- T_387737843__/RConn3 -- bus113/LConn1
  T_296560688__/RConn1 -- L_296560688/LConn1
  T_296560688__/RConn2 -- L_296560688/LConn2
  L_296560688/LConn3 -- T_296560688__/RConn3 -- bus114/LConn1
  T_404291513__/RConn1 -- L_404291513/LConn1
  T_404291513__/RConn2 -- L_404291513/LConn2
  L_404291513/LConn3 -- T_404291513__/RConn3 -- bus115/LConn1
  T_64680223_230000_/RConn1 -- L_64680223/LConn1
  T_64680223_230000_/RConn2 -- L_64680223/LConn2
  L_64680223/LConn3 -- T_64680223_230000_/RConn3 -- bus116/LConn1
  T_345996520__/RConn1 -- L_345996520/LConn1
  T_345996520__/RConn2 -- L_345996520/LConn2
  L_345996520/LConn3 -- T_345996520__/RConn3 -- bus117/LConn1
  T_324258748__HVDC_Thai__Mal/RConn1 -- L_324258748/LConn1
  T_324258748__HVDC_Thai__Mal/RConn2 -- L_324258748/LConn2
  L_324258748/LConn3 -- T_324258748__HVDC_Thai__Mal/RConn3 -- bus118/LConn1
  T_144455497__/RConn1 -- L_144455497/LConn1
  T_144455497__/RConn2 -- L_144455497/LConn2
  L_144455497/LConn3 -- T_144455497__/RConn3 -- bus119/LConn1
  T_64680159__/RConn1 -- L_64680159/LConn1
  T_64680159__/RConn2 -- L_64680159/LConn2
  L_64680159/LConn3 -- T_64680159__/RConn3 -- bus120/LConn1
  T_381850832_230000;115000_Phangnga/RConn1 -- L_381850832/LConn1
  T_381850832_230000;115000_Phangnga/RConn2 -- L_381850832/LConn2
  L_381850832/LConn3 -- T_381850832_230000;115000_Phangnga/RConn3 -- bus121/LConn1
  T_381850842_230000;115000_Phuket_2/RConn1 -- L_381850842/LConn1
  T_381850842_230000;115000_Phuket_2/RConn2 -- L_381850842/LConn2
  L_381850842/LConn3 -- T_381850842_230000;115000_Phuket_2/RConn3 -- bus122/LConn1
  T_384684882__/RConn1 -- L_384684882/LConn1
  T_384684882__/RConn2 -- L_384684882/LConn2
  L_384684882/LConn3 -- T_384684882__/RConn3 -- bus123/LConn1
  T_293324904__/RConn1 -- L_293324904/LConn1
  T_293324904__/RConn2 -- L_293324904/LConn2
  L_293324904/LConn3 -- T_293324904__/RConn3 -- bus124/LConn1
  T_293324915__/RConn1 -- L_293324915/LConn1
  T_293324915__/RConn2 -- L_293324915/LConn2
  L_293324915/LConn3 -- T_293324915__/RConn3 -- bus125/LConn1
  T_242402501__/RConn1 -- L_242402501/LConn1
  T_242402501__/RConn2 -- L_242402501/LConn2
  L_242402501/LConn3 -- T_242402501__/RConn3 -- bus126/LConn1
  T_362353137__/RConn1 -- L_362353137/LConn1
  T_362353137__/RConn2 -- L_362353137/LConn2
  L_362353137/LConn3 -- T_362353137__/RConn3 -- bus127/LConn1
  T_261489769_500000_/RConn1 -- L_261489769/LConn1
  T_261489769_500000_/RConn2 -- L_261489769/LConn2
  L_261489769/LConn3 -- T_261489769_500000_/RConn3 -- bus128/LConn1
